simulink model "DMC_simulink_trial_2_SISO"  (R2015a)
settings: Solver=ode45  StartTime=0.0  StopTime=60  RelTol=1e-3
values from neighbouring files (symbols this model uses):
  Fac = (inv(G'*G+lambda*eye(2*(M+1))))*(G')    [DMC_MIMO_DATA_Gen.m]    (also in DMC_SISO_DATA_Gen.m = (inv(G'*G+lambda*eye(M+1)))*(G'))
  temp_f = [temp_f_11 temp_f_12;temp_f_21 temp_f_22]    [DMC_MIMO_DATA_Gen.m]    (also in DMC_SISO_DATA_Gen.m = temp_g1 - temp_g2)
settings Model: Creator=Ronak  LastModifiedBy=Ronak

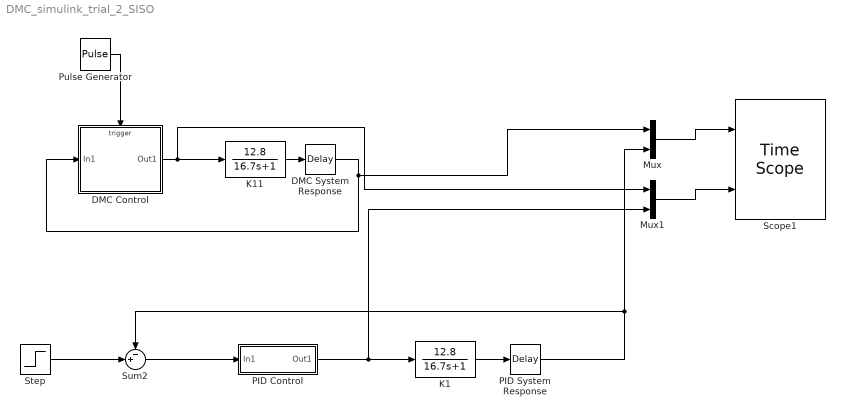
== system DMC_simulink_trial_2_SISO ==
  DMC Control : Subsystem  TreatAsAtomicUnit=on
  DMC System Response : TransportDelay
  K1 : TransferFcn  Numerator=[12.8]  Denominator=[16.7 1]
  K11 : TransferFcn  Numerator=[12.8]  Denominator=[16.7 1]
  Mux : Mux  Inputs=2
  Mux1 : Mux  Inputs=2
  PID Control : Subsystem
  PID System Response : TransportDelay
  Pulse Generator : DiscretePulseGenerator  PulseType=Time based  Period=0.1  PulseWidth=5
  Scope1 : TimeScope  NumInputPorts=2
  Step : Step  After=10  SampleTime=0
  Sum2 : Sum  Inputs=-+|
  wires:
  K11/1 -> DMC System Response/1
  Pulse Generator/1 -> DMC Control/Trigger
  DMC Control/1(Out1) -> Mux1/1, K11/1
  DMC System Response/1 -> Mux/1, DMC Control/1(In1)
  K1/1 -> PID System Response/1
  PID Control/1(Out1) -> Mux1/2, K1/1
  PID System Response/1 -> Mux/2, Sum2/1
  Sum2/1 -> PID Control/1(In1)
  Step/1 -> Sum2/2
  Mux/1 -> Scope1/1
  Mux1/1 -> Scope1/2

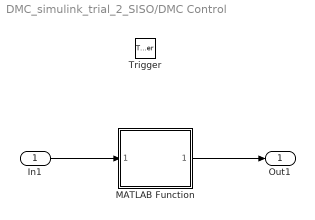
== system DMC_simulink_trial_2_SISO/DMC Control ==
  In1 : Inport
  Trigger : TriggerPort
  MATLAB Function : MATLAB Function  TreatAsAtomicUnit=on
  Out1 : Outport
  wires:
  MATLAB Function/1(u_optimal) -> Out1/1
  In1/1 -> MATLAB Function/1(y_meas)

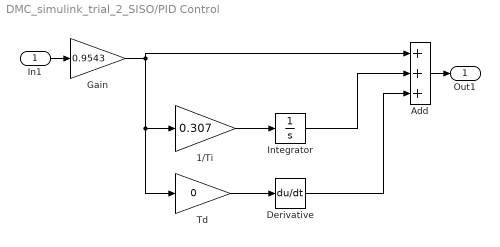
== system DMC_simulink_trial_2_SISO/PID Control ==
  In1 : Inport
  1/Ti : Gain  Gain=0.307
  Add : Sum  Inputs=+++
  Derivative : Derivative
  Gain : Gain  Gain=0.9543
  Integrator : Integrator
  Td : Gain  Gain=0
  Out1 : Outport
  wires:
  In1/1 -> Gain/1
  Add/1 -> Out1/1
  Gain/1 -> Add/1, Td/1, 1/Ti/1
  Integrator/1 -> Add/2
  Derivative/1 -> Add/3
  1/Ti/1 -> Integrator/1
  Td/1 -> Derivative/1

== matlab function DMC_simulink_trial_2_SISO/DMC Control/MATLAB Function ==
  data: y_meas input; u_optimal output; Fac parameter; temp_f parameter
function u_optimal = fcn(y_meas,Fac,temp_f)
%#codegen
coder.extrinsic('evalin', 'assignin')
r = y_meas;
y_sp = 10;
u = zeros(1700,1);  % here in triggered system zeros(N,1) is giving error
u = evalin('base','u'); % Read value from workspace
u_old = 0;
u_old = evalin('base','u_old'); 
alpha = 0.9; 
ref = zeros(1,600);
for i =1:600
    r = alpha*r + (1-alpha)*y_sp;
    ref(i) = r;
end
f = y_meas*ones(600,1);
f = f + temp_f*u;
u_temp = Fac*(ref'-f);
u_optimal = u_old + u_temp(1);
u = [u_temp(1);u(1:end-1,1)];
assignin('base','u',u);
assignin('base','u_old',u_optimal);
end
